simulink library "INT_MeUn_DD"  (R2016b)
settings: Solver=VariableStepAuto  StartTime=0.0  StopTime=10.0  RelTol=1e-3
settings Model: Creator=liutao  LastModifiedBy=liutao

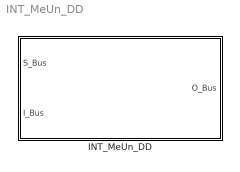
== system INT_MeUn_DD ==
  INT_MeUn_DD : Subsystem

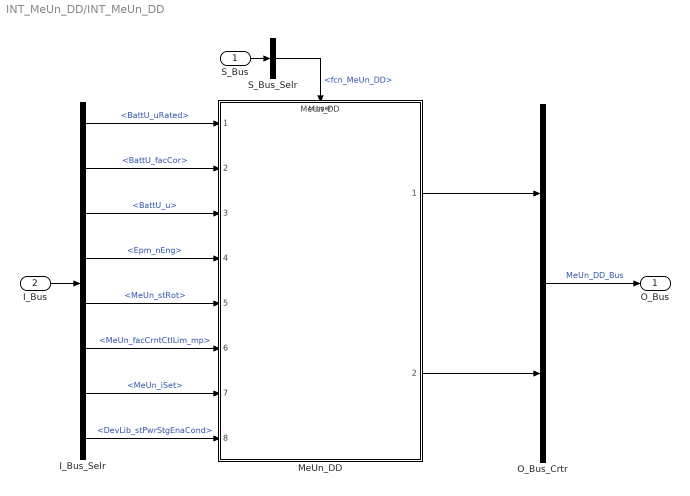
== system INT_MeUn_DD/INT_MeUn_DD ==
  S_Bus : Inport
  I_Bus : Inport  Port=2
  I_Bus_Selr : BusSelector  OutputSignals=BattU_uRated,BattU_facCor,BattU_u,Epm_nEng,MeUn_stRot,MeUn_facCrntCtlLim_mp,MeUn_iSet,DevLib_stPwrStgEnaCond
  MeUn_DD : ModelReference  ModelNameDialog=MeUn_DD  SimulationMode=Normal  ModelReferenceVersion=1.26  TriggerPortName=function  TriggerPortTriggerType=function-call  TriggerPortStatesWhenEnabling=held
  O_Bus_Crtr : BusCreator  Inputs=2
  S_Bus_Selr : BusSelector  OutputSignals=fcn_MeUn_DD
  O_Bus : Outport
  wires:
  S_Bus_Selr/1 -> MeUn_DD/Trigger  "<fcn_MeUn_DD>"
  S_Bus/1 -> S_Bus_Selr/1
  I_Bus/1 -> I_Bus_Selr/1
  I_Bus_Selr/1 -> MeUn_DD/1  "<BattU_uRated>"
  I_Bus_Selr/2 -> MeUn_DD/2  "<BattU_facCor>"
  I_Bus_Selr/3 -> MeUn_DD/3  "<BattU_u>"
  I_Bus_Selr/4 -> MeUn_DD/4  "<Epm_nEng>"
  I_Bus_Selr/5 -> MeUn_DD/5  "<MeUn_stRot>"
  I_Bus_Selr/6 -> MeUn_DD/6  "<MeUn_facCrntCtlLim_mp>"
  I_Bus_Selr/7 -> MeUn_DD/7  "<MeUn_iSet>"
  I_Bus_Selr/8 -> MeUn_DD/8  "<DevLib_stPwrStgEnaCond>"
  O_Bus_Crtr/1 -> O_Bus/1  "MeUn_DD_Bus"
  MeUn_DD/1 -> O_Bus_Crtr/1
  MeUn_DD/2 -> O_Bus_Crtr/2
